simulink model "P2_Indirect_force_control"  (Simulink 9.3)
settings: Solver=ode23  StartTime=0.0  StopTime=t_d  MaxStep=Tc  RelTol=1e-8  AbsTol=1e-8
values from neighbouring files (symbols this model uses):
  F_v = K_r*diag([0.01 0.01])*K_r    [init_2.m]
  g = 9.81    [init_2.m]
  K_d = 500*diag([1 1])    [init_2.m]
  K_p = 16250*diag([1 1])    [init_2.m]
  oe = [(K_p(1)*x_d(1) + K(1)*or(1))/(K_p(1) + K(1)) x_d(2)]'    [init_2.m]
  pi_l = pi_m    [init_2.m]
  q_i = [0 pi/5]    [init_2.m]
  Tc = 0.001    [init_2.m]
  Ts = Tc    (= 0.001)    [init_2.m]
undefined symbols (not defined in the file or in its folder): a, fkine_2p, iner_l, jacob_2p
settings Model: Creator=luigivillani  LastModifiedBy=Ravi Pipaliya  ExtModeAutoUpdateStatusClock=off
settings SolverCC: AutoScaleAbsTol=off  InitialStep=0.1*Tc
settings DataIOCC: SaveOutput=off  SaveTime=off
settings OptimizationCC: BlockReduction=off  BooleanDataType=off  ExpressionDepthLimit=2147483647  InitFltsAndDblsToZero=on
settings DebuggingCC: SaveWithParameterizedLinksMsg=none  SignalResolutionControl=TryResolveAllWithWarning  MultiTaskDSMMsg=warning  MultiTaskCondExecSysMsg=none  StateNameClashWarn=warning
settings HardwareCC: TargetUnknown=on
settings SFSimCC: SimUseLocalCustomCode=on
settings RTWCC: RTWUseLocalCustomCode=on
settings GRTTargetCC: TargetFcnLib=ansi_tfl_tmw.mat
settings ConfigComp: CovExternalEMLEnable=on

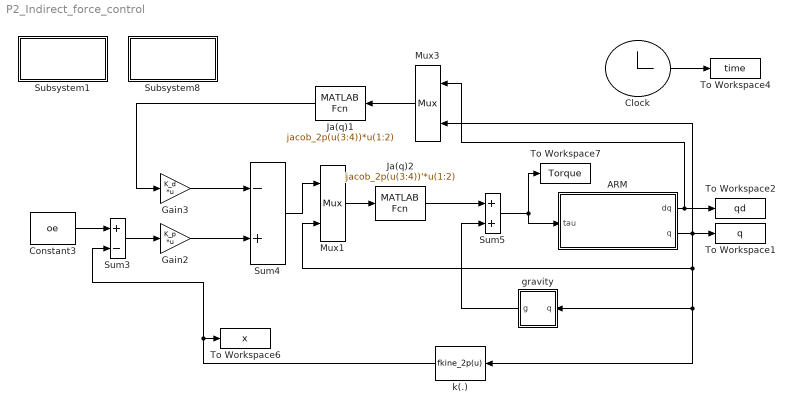
== system P2_Indirect_force_control ==
  ARM : Subsystem
      mask Display: disp('MANIPULATOR')
  Clock : Clock
  Constant3 : Constant  Value=oe
      mask Display: disp('x_d')
  Gain2 : Gain  Gain=K_p  Multiplication=Matrix(K*u)  SampleTime=Tc
      mask Display: disp('K_p')
  Gain3 : Gain  Gain=K_d  Multiplication=Matrix(K*u)  SampleTime=Tc
      mask Display: disp('K_d')
  Ja(q)1 : MATLABFcn  MATLABFcn=jacob_2p(u(3:4))*u(1:2)  OutputDimensions=2
      mask Display: disp('Ja(q)')
  Ja(q)2 : MATLABFcn  MATLABFcn=jacob_2p(u(3:4))'*u(1:2)  OutputDimensions=2
      mask Display: disp("Ja(q)'")
  Mux1 : Mux  Inputs=[2,2]
  Mux3 : Mux  Inputs=[2,2]
  Subsystem1 : Subsystem
      settings: OpenFcn=init_2;  ErrorFcn=init_1
      mask Display: disp('Initialize')
  Subsystem8 : Subsystem
      settings: OpenFcn=plot_2;  ErrorFcn=plot_1
      mask Display: disp('Plot Output')
  Sum3 : Sum  Inputs=+-  SampleTime=Tc  SaturateOnIntegerOverflow=on  InputSameDT=on  OutDataTypeStr=Inherit: Same as first input
  Sum4 : Sum  Inputs=-+  SaturateOnIntegerOverflow=on  InputSameDT=on  OutDataTypeStr=Inherit: Same as first input
  Sum5 : Sum  SampleTime=Tc  SaturateOnIntegerOverflow=on  InputSameDT=on  OutDataTypeStr=Inherit: Same as first input
  To Workspace1 : ToWorkspace  VariableName=q  SampleTime=Ts
      settings: MaxDataPoints=4001
  To Workspace2 : ToWorkspace  VariableName=qd  SampleTime=Ts
      settings: MaxDataPoints=4001
  To Workspace4 : ToWorkspace  VariableName=time  SampleTime=Ts
      settings: MaxDataPoints=4001
  To Workspace6 : ToWorkspace  VariableName=x  SampleTime=Ts
      settings: MaxDataPoints=4001
  To Workspace7 : ToWorkspace  VariableName=Torque  SampleTime=Ts
      settings: MaxDataPoints=4001
  gravity : Subsystem
      mask Display: disp('g(q)')
  "k(.) " : MATLABFcn  MATLABFcn=fkine_2p(u)  OutputDimensions=2
      mask Display: disp('k(.)')
  wires:
  Clock/1 -> To Workspace4/1
  Sum3/1 -> Gain2/1
  Constant3/1 -> Sum3/1
  ARM/1(dq) -> Mux3/1, To Workspace2/1
  "k(.) "/1 -> Sum3/2, To Workspace6/1
  Sum5/1 -> ARM/1(tau), To Workspace7/1
  gravity/1(g) -> Sum5/2
  Gain2/1 -> Sum4/2
  Gain3/1 -> Sum4/1
  Ja(q)1/1 -> Gain3/1
  Mux3/1 -> Ja(q)1/1
  Ja(q)2/1 -> Sum5/1
  Sum4/1 -> Mux1/1
  ARM/2("q ") -> Mux3/2, Mux1/2, "k(.) "/1, gravity/1(q), To Workspace1/1
  Mux1/1 -> Ja(q)2/1

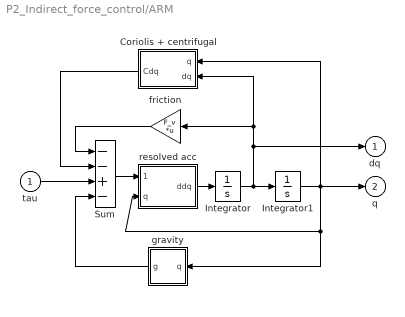
== system P2_Indirect_force_control/ARM ==
  tau : Inport
  Coriolis + centrifugal : Subsystem
      mask Display: disp('C(q,dq)dq')
  Integrator : Integrator  InitialCondition=[0 0]  ZeroCross=off
  Integrator1 : Integrator  InitialCondition=q_i  ZeroCross=off
  Sum : Sum  Inputs=--+-  SaturateOnIntegerOverflow=on  InputSameDT=on  OutDataTypeStr=Inherit: Same as first input
  friction : Gain  Gain=F_v  Multiplication=Matrix(K*u)  SaturateOnIntegerOverflow=on  OutDataTypeStr=Inherit: Same as input  ParamDataTypeStr=Inherit: Same as input
      mask Display: disp('F_v')
  gravity : Subsystem
      mask Display: disp('g(q)')
  resolved acc : Subsystem
      mask Display: disp('inv(B(q))')
  dq : Outport  InitialOutput=0
  "q " : Outport  Port=2  InitialOutput=0
  wires:
  Coriolis + centrifugal/1(Cdq) -> Sum/2
  tau/1 -> Sum/3
  Integrator1/1 -> Coriolis + centrifugal/1(q), resolved acc/2(q), gravity/1(q), "q "/1
  resolved acc/1(ddq) -> Integrator/1
  Integrator/1 -> Integrator1/1, dq/1, Coriolis + centrifugal/2(dq), friction/1
  Sum/1 -> resolved acc/1(tau-tau')
  friction/1 -> Sum/1
  gravity/1(g) -> Sum/4

== system P2_Indirect_force_control/Subsystem1 ==
  note: start

== system P2_Indirect_force_control/Subsystem8 ==
  note: start

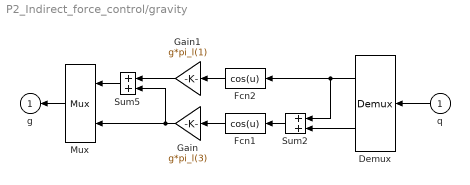
== system P2_Indirect_force_control/gravity ==
  q : Inport
  Demux : Demux  Outputs=2
  Fcn1 : Fcn  Expr=cos(u)
  Fcn2 : Fcn  Expr=cos(u)
  Gain : Gain  Gain=g*pi_l(3)  SaturateOnIntegerOverflow=on  OutDataTypeStr=Inherit: Same as input  ParamDataTypeStr=Inherit: Same as input
      mask Display: disp('k_2')
  Gain1 : Gain  Gain=g*pi_l(1)  SaturateOnIntegerOverflow=on  OutDataTypeStr=Inherit: Same as input  ParamDataTypeStr=Inherit: Same as input
      mask Display: disp('k_1')
  Mux : Mux  Inputs=2
  Sum2 : Sum  SaturateOnIntegerOverflow=on  InputSameDT=on  OutDataTypeStr=Inherit: Same as first input
  Sum5 : Sum  SaturateOnIntegerOverflow=on  InputSameDT=on  OutDataTypeStr=Inherit: Same as first input
  g : Outport  InitialOutput=0
  wires:
  q/1 -> Demux/1
  Demux/2 -> Sum2/2
  Sum2/1 -> Fcn1/1
  Fcn1/1 -> Gain/1
  Fcn2/1 -> Gain1/1
  Demux/1 -> Fcn2/1, Sum2/1
  Gain1/1 -> Sum5/1
  Sum5/1 -> Mux/1
  Gain/1 -> Sum5/2, Mux/2
  Mux/1 -> g/1

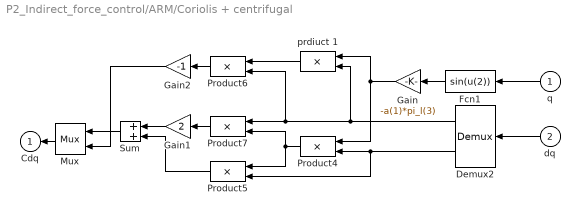
== system P2_Indirect_force_control/ARM/Coriolis + centrifugal ==
  q : Inport
  dq : Inport  Port=2
  Demux2 : Demux  Outputs=2
  Fcn1 : Fcn  Expr=sin(u(2))
  Gain : Gain  Gain=-a(1)*pi_l(3)  SaturateOnIntegerOverflow=on  OutDataTypeStr=Inherit: Same as input  ParamDataTypeStr=Inherit: Same as input
      mask Display: disp('k_3')
  Gain1 : Gain  Gain=2  SaturateOnIntegerOverflow=on  OutDataTypeStr=Inherit: Same as input  ParamDataTypeStr=Inherit: Same as input
  Gain2 : Gain  Gain=-1  SaturateOnIntegerOverflow=on  OutDataTypeStr=Inherit: Same as input  ParamDataTypeStr=Inherit: Same as input
  Mux : Mux  Inputs=2
  Product{4..7} (4 alike) : Product  SaturateOnIntegerOverflow=on  RndMeth=Zero  InputSameDT=on  OutDataTypeStr=Inherit: Same as first input
  Sum : Sum  SaturateOnIntegerOverflow=on  InputSameDT=on  OutDataTypeStr=Inherit: Same as first input
  prdiuct 1 : Product  SaturateOnIntegerOverflow=on  RndMeth=Zero  InputSameDT=on  OutDataTypeStr=Inherit: Same as first input
  Cdq : Outport  InitialOutput=0
  wires:
  dq/1 -> Demux2/1
  Gain2/1 -> Mux/2
  Product6/1 -> Gain2/1
  Mux/1 -> Cdq/1
  Sum/1 -> Mux/1
  Product5/1 -> Sum/2
  Gain1/1 -> Sum/1
  Product7/1 -> Gain1/1
  Demux2/1 -> prdiuct 1/2, Product6/2, Product7/1
  Demux2/2 -> Product4/2, Product5/2
  prdiuct 1/1 -> Product6/1
  Gain/1 -> prdiuct 1/1, Product4/1
  Fcn1/1 -> Gain/1
  q/1 -> Fcn1/1
  Product4/1 -> Product5/1, Product7/2

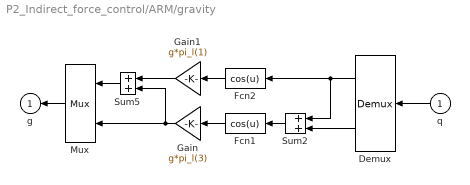
== system P2_Indirect_force_control/ARM/gravity ==
  q : Inport
  Demux : Demux  Outputs=2
  Fcn1 : Fcn  Expr=cos(u)
  Fcn2 : Fcn  Expr=cos(u)
  Gain : Gain  Gain=g*pi_l(3)  SaturateOnIntegerOverflow=on  OutDataTypeStr=Inherit: Same as input  ParamDataTypeStr=Inherit: Same as input
      mask Display: disp('k_2')
  Gain1 : Gain  Gain=g*pi_l(1)  SaturateOnIntegerOverflow=on  OutDataTypeStr=Inherit: Same as input  ParamDataTypeStr=Inherit: Same as input
      mask Display: disp('k_1')
  Mux : Mux  Inputs=2
  Sum2 : Sum  SaturateOnIntegerOverflow=on  InputSameDT=on  OutDataTypeStr=Inherit: Same as first input
  Sum5 : Sum  SaturateOnIntegerOverflow=on  InputSameDT=on  OutDataTypeStr=Inherit: Same as first input
  g : Outport  InitialOutput=0
  wires:
  q/1 -> Demux/1
  Demux/2 -> Sum2/2
  Sum2/1 -> Fcn1/1
  Fcn1/1 -> Gain/1
  Fcn2/1 -> Gain1/1
  Demux/1 -> Fcn2/1, Sum2/1
  Gain1/1 -> Sum5/1
  Sum5/1 -> Mux/1
  Gain/1 -> Sum5/2, Mux/2
  Mux/1 -> g/1

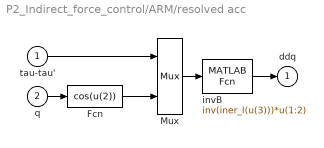
== system P2_Indirect_force_control/ARM/resolved acc ==
  tau-tau' : Inport
  q : Inport  Port=2
  Fcn : Fcn  Expr=cos(u(2))
  Mux : Mux  Inputs=[2,1]
  "invB " : MATLABFcn  MATLABFcn=inv(iner_l(u(3)))*u(1:2)  OutputDimensions=2
      mask Display: disp('inv(B(q))')
  ddq : Outport  InitialOutput=0
  wires:
  Fcn/1 -> Mux/2
  q/1 -> Fcn/1
  "invB "/1 -> ddq/1
  tau-tau'/1 -> Mux/1
  Mux/1 -> "invB "/1
